simulink model "KE_time"  (Simulink 7.9)
settings: Solver=ode14x  StartTime=0.0  StopTime=6.6  FixedStep=Tsamp  RelTol=Tsamp
values from neighbouring files (symbols this model uses):
  A_hat = A_maglev    [Initialise_LQG_observers_igva.m]
  B_hat = B_maglev(:,2)    [Initialise_LQG_observers_igva.m]
  C_hat_ga = C_maglev(sensors_selected,:)    [Initialise_LQG_observers_igva.m]
  C_hat_gv = C_maglev(sensors_selected,:)    [Initialise_LQG_observers_igva.m]
  C_hat_gva = C_maglev(sensors_selected,:)    [Initialise_LQG_observers_igva.m]
  C_hat_ig = C_maglev(sensors_selected,:)    [Initialise_LQG_observers_igva.m]
  C_hat_iga = C_maglev(sensors_selected,:)    [Initialise_LQG_observers_igva.m]
  C_hat_igv = C_maglev(sensors_selected,:)    [Initialise_LQG_observers_igva.m]
  C_hat_igva = C_maglev(sensors_selected,:)    [Initialise_LQG_observers_igva.m]
  D_hat_ga = D_maglev(sensors_selected,1)    [Initialise_LQG_observers_igva.m]
  D_hat_gv = D_maglev(sensors_selected,1)    [Initialise_LQG_observers_igva.m]
  D_hat_gva = D_maglev(sensors_selected,1)    [Initialise_LQG_observers_igva.m]
  D_hat_ig = D_maglev(sensors_selected,1)    [Initialise_LQG_observers_igva.m]
  D_hat_iga = D_maglev(sensors_selected,1)    [Initialise_LQG_observers_igva.m]
  D_hat_igv = D_maglev(sensors_selected,1)    [Initialise_LQG_observers_igva.m]
  D_hat_igva = D_maglev(sensors_selected,1)    [Initialise_LQG_observers_igva.m]
  sensor_matrix_ga = sensor_matrix_full(sensors_selected,:)    [Initialise_LQG_observers_igva.m]    (also in LSDP_controllers_nntraining_data_igva.m = sensors(sensor_sele,:); initialize_LSDP_controllers_igva.m = sensors(sensor_sele,:))
  sensor_matrix_gv = sensor_matrix_full(sensors_selected,:)    [Initialise_LQG_observers_igva.m]    (also in LSDP_controllers_nntraining_data_igva.m = sensors(sensor_sele,:); initialize_LSDP_controllers_igva.m = sensors(sensor_sele,:))
  sensor_matrix_gva = sensor_matrix_full(sensors_selected,:)    [Initialise_LQG_observers_igva.m]    (also in LSDP_controllers_nntraining_data_igva.m = sensors(sensor_sele,:); initialize_LSDP_controllers_igva.m = sensors(sensor_sele,:))
  sensor_matrix_ig = sensor_matrix_full(sensors_selected,:)    [Initialise_LQG_observers_igva.m]    (also in LSDP_controllers_nntraining_data_igva.m = sensors(sensor_sele,:); initialize_LSDP_controllers_igva.m = sensors(sensor_sele,:))
  sensor_matrix_iga = sensor_matrix_full(sensors_selected,:)    [Initialise_LQG_observers_igva.m]    (also in initialize_LSDP_controllers_igva.m = sensors(sensor_sele,:))
  sensor_matrix_igv = sensor_matrix_full(sensors_selected,:)    [Initialise_LQG_observers_igva.m]    (also in LSDP_controllers_nntraining_data_igva.m = sensors(sensor_sele,:); initialize_LSDP_controllers_igva.m = sensors(sensor_sele,:))
  sensor_matrix_igva = sensors(sensor_sele,:)    [LSDP_controllers_nntraining_data_igva.m]    (also in initialize_LSDP_controllers_igva.m)
undefined symbols (not defined in the file or in its folder): Kf_lqg_ga, Kf_lqg_gv, Kf_lqg_gva, Kf_lqg_ig, Kf_lqg_iga, Kf_lqg_igv, Kf_lqg_igva
settings Model: Creator=kostas  LastModifiedBy=kostas

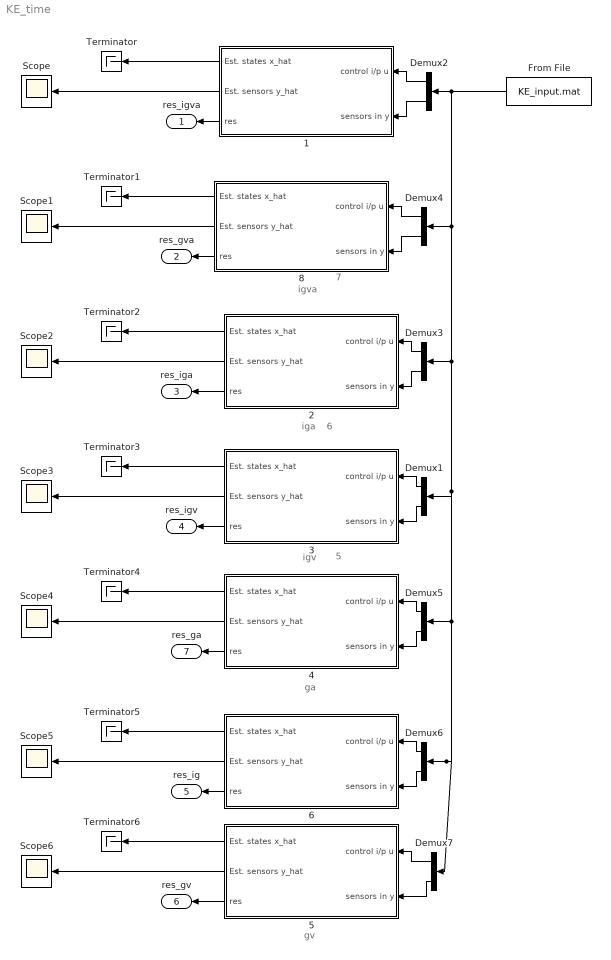
== system KE_time ==
  note: igva
  note: iga
  note: igv
  note: ga
  note: gv
  note: 7
  note: 6
  note: 5
  " 1" : Subsystem
      mask Display: fprintf('\n\n Kalman Bucy Filter \n\n (Continuous Time)\n\n')
  " 2" : Subsystem
      mask Display: fprintf('\n\n Kalman Bucy Filter \n\n (Continuous Time)\n\n')
  " 3" : Subsystem
      mask Display: fprintf('\n\n Kalman Bucy Filter \n\n (Continuous Time)\n\n')
  " 4" : Subsystem
      mask Display: fprintf('\n\n Kalman Bucy Filter \n\n (Continuous Time)\n\n')
  " 5" : Subsystem
      mask Display: fprintf('\n\n Kalman Bucy Filter \n\n (Continuous Time)\n\n')
  " 6" : Subsystem
      mask Display: fprintf('\n\n Kalman Bucy Filter \n\n (Continuous Time)\n\n')
  " 8" : Subsystem
      mask Display: fprintf('\n\n Kalman Bucy Filter \n\n (Continuous Time)\n\n')
  Demux{1..7} (7 alike) : Demux  Outputs=2
  From File : FromFile  FileName=KE_input.mat  SampleTime=0
  Scope{,1..6} (7 alike) : Scope
      Scope2 settings: SaveName=ScopeData2
      Scope3 settings: SaveName=ScopeData3
      Scope4 settings: SaveName=ScopeData4
      Scope5 settings: SaveName=ScopeData5
      Scope6 settings: SaveName=ScopeData6
  Terminator{,1..6} (7 alike) : Terminator
  res_igva : Outport
  res_gva : Outport  Port=2
  res_iga : Outport  Port=3
  res_igv : Outport  Port=4
  res_ig : Outport  Port=5
  res_gv : Outport  Port=6
  res_ga : Outport  Port=7
  wires:
  Demux2/1 -> " 1"/1(control i/p u)
  Demux2/2 -> " 1"/2(" sensors in y")
  Demux3/1 -> " 2"/1(control i/p u)
  Demux3/2 -> " 2"/2(" sensors in y")
  Demux1/1 -> " 3"/1(control i/p u)
  Demux1/2 -> " 3"/2(" sensors in y")
  Demux5/1 -> " 4"/1(control i/p u)
  Demux5/2 -> " 4"/2(" sensors in y")
  Demux6/1 -> " 6"/1(control i/p u)
  Demux6/2 -> " 6"/2(" sensors in y")
  Demux7/1 -> " 5"/1(control i/p u)
  Demux7/2 -> " 5"/2(" sensors in y")
  " 1"/3(res) -> res_igva/1
  " 2"/3(res) -> res_iga/1
  " 3"/3(res) -> res_igv/1
  " 4"/3(res) -> res_ga/1
  " 6"/3(res) -> res_ig/1
  " 5"/3(res) -> res_gv/1
  Demux4/1 -> " 8"/1(control i/p u)
  Demux4/2 -> " 8"/2(" sensors in y")
  " 8"/3(res) -> res_gva/1
  From File/1 -> Demux2/1, Demux4/1, Demux3/1, Demux5/1, Demux6/1, Demux7/1, Demux1/1
  " 1"/2(Est. sensors y_hat) -> Scope/1
  " 8"/2(Est. sensors y_hat) -> Scope1/1
  " 2"/2(Est. sensors y_hat) -> Scope2/1
  " 3"/2(Est. sensors y_hat) -> Scope3/1
  " 4"/2(Est. sensors y_hat) -> Scope4/1
  " 6"/2(Est. sensors y_hat) -> Scope5/1
  " 5"/2(Est. sensors y_hat) -> Scope6/1
  " 1"/1(Est. states x_hat) -> Terminator/1
  " 8"/1(Est. states x_hat) -> Terminator1/1
  " 2"/1(Est. states x_hat) -> Terminator2/1
  " 3"/1(Est. states x_hat) -> Terminator3/1
  " 4"/1(Est. states x_hat) -> Terminator4/1
  " 6"/1(Est. states x_hat) -> Terminator5/1
  " 5"/1(Est. states x_hat) -> Terminator6/1

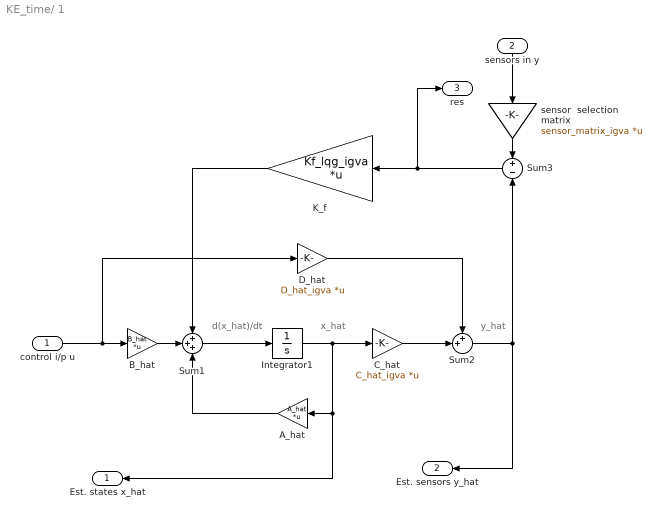
== system KE_time/ 1 ==
  note: d(x_hat)/dt
  note: x_hat
  note: y_hat
  control i/p u : Inport
  " sensors in y" : Inport  Port=2
  "A_hat " : Gain  Gain=A_hat  Multiplication=Matrix(K*u)  SaturateOnIntegerOverflow=on  OutDataTypeStr=Inherit: Same as input  ParamDataTypeStr=Inherit: Same as input
  B_hat : Gain  Gain=B_hat  Multiplication=Matrix(K*u)  SaturateOnIntegerOverflow=on  OutDataTypeStr=Inherit: Same as input  ParamDataTypeStr=Inherit: Same as input
  C_hat : Gain  Gain=C_hat_igva  Multiplication=Matrix(K*u)  SaturateOnIntegerOverflow=on  OutDataTypeStr=Inherit: Same as input  ParamDataTypeStr=Inherit: Same as input
  D_hat : Gain  Gain=D_hat_igva  Multiplication=Matrix(K*u)  SaturateOnIntegerOverflow=on  OutDataTypeStr=Inherit: Same as input  ParamDataTypeStr=Inherit: Same as input
  Integrator1 : Integrator
  K_f : Gain  Gain=Kf_lqg_igva  Multiplication=Matrix(K*u)  SaturateOnIntegerOverflow=on  OutDataTypeStr=Inherit: Same as input  ParamDataTypeStr=Inherit: Same as input
  Sum1 : Sum  Inputs=+++  SaturateOnIntegerOverflow=on  InputSameDT=on  OutDataTypeStr=Inherit: Same as first input
  Sum2 : Sum  Inputs=++|  SaturateOnIntegerOverflow=on  InputSameDT=on  OutDataTypeStr=Inherit: Same as first input
  Sum3 : Sum  Inputs=+|-  SaturateOnIntegerOverflow=on  InputSameDT=on  OutDataTypeStr=Inherit: Same as first input
  sensor  selection  matrix : Gain  Gain=sensor_matrix_igva  Multiplication=Matrix(K*u) (u vector)
  Est. states x_hat : Outport  OutputWhenDisabled=reset  InitialOutput=[0 0 0]
  Est. sensors y_hat : Outport  Port=2
  res : Outport  Port=3
  wires:
  Sum2/1 -> Est. sensors y_hat/1, Sum3/2
  D_hat/1 -> Sum2/1
  C_hat/1 -> Sum2/2
  control i/p u/1 -> D_hat/1, B_hat/1
  " sensors in y"/1 -> sensor  selection  matrix/1
  Sum3/1 -> K_f/1, res/1
  K_f/1 -> Sum1/1
  Integrator1/1 -> Est. states x_hat/1, "A_hat "/1, C_hat/1
  Sum1/1 -> Integrator1/1
  "A_hat "/1 -> Sum1/3
  B_hat/1 -> Sum1/2
  sensor  selection  matrix/1 -> Sum3/1

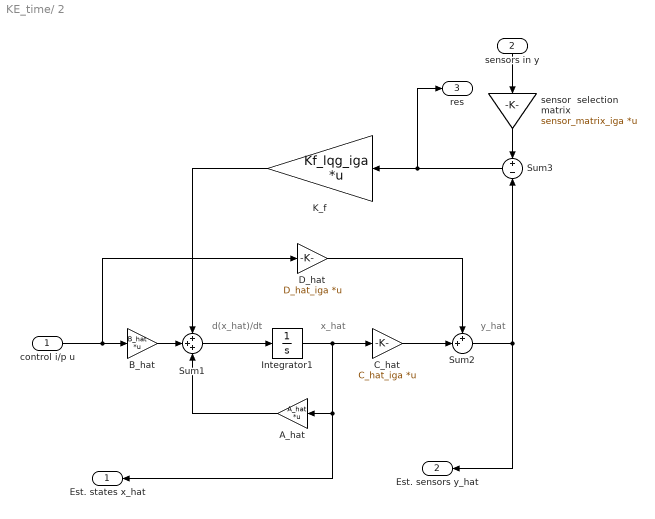
== system KE_time/ 2 ==
  note: y_hat
  note: x_hat
  note: d(x_hat)/dt
  control i/p u : Inport
  " sensors in y" : Inport  Port=2
  "A_hat " : Gain  Gain=A_hat  Multiplication=Matrix(K*u)  SaturateOnIntegerOverflow=on  OutDataTypeStr=Inherit: Same as input  ParamDataTypeStr=Inherit: Same as input
  B_hat : Gain  Gain=B_hat  Multiplication=Matrix(K*u)  SaturateOnIntegerOverflow=on  OutDataTypeStr=Inherit: Same as input  ParamDataTypeStr=Inherit: Same as input
  C_hat : Gain  Gain=C_hat_iga  Multiplication=Matrix(K*u)  SaturateOnIntegerOverflow=on  OutDataTypeStr=Inherit: Same as input  ParamDataTypeStr=Inherit: Same as input
  D_hat : Gain  Gain=D_hat_iga  Multiplication=Matrix(K*u)  SaturateOnIntegerOverflow=on  OutDataTypeStr=Inherit: Same as input  ParamDataTypeStr=Inherit: Same as input
  Integrator1 : Integrator
  K_f : Gain  Gain=Kf_lqg_iga  Multiplication=Matrix(K*u)  SaturateOnIntegerOverflow=on  OutDataTypeStr=Inherit: Same as input  ParamDataTypeStr=Inherit: Same as input
  Sum1 : Sum  Inputs=+++  SaturateOnIntegerOverflow=on  InputSameDT=on  OutDataTypeStr=Inherit: Same as first input
  Sum2 : Sum  Inputs=++|  SaturateOnIntegerOverflow=on  InputSameDT=on  OutDataTypeStr=Inherit: Same as first input
  Sum3 : Sum  Inputs=+|-  SaturateOnIntegerOverflow=on  InputSameDT=on  OutDataTypeStr=Inherit: Same as first input
  sensor  selection  matrix : Gain  Gain=sensor_matrix_iga  Multiplication=Matrix(K*u) (u vector)
  Est. states x_hat : Outport  OutputWhenDisabled=reset  InitialOutput=[0 0 0]
  Est. sensors y_hat : Outport  Port=2
  res : Outport  Port=3
  wires:
  sensor  selection  matrix/1 -> Sum3/1
  B_hat/1 -> Sum1/2
  "A_hat "/1 -> Sum1/3
  Sum1/1 -> Integrator1/1
  Integrator1/1 -> C_hat/1, "A_hat "/1, Est. states x_hat/1
  K_f/1 -> Sum1/1
  Sum3/1 -> K_f/1, res/1
  " sensors in y"/1 -> sensor  selection  matrix/1
  control i/p u/1 -> B_hat/1, D_hat/1
  C_hat/1 -> Sum2/2
  D_hat/1 -> Sum2/1
  Sum2/1 -> Sum3/2, Est. sensors y_hat/1

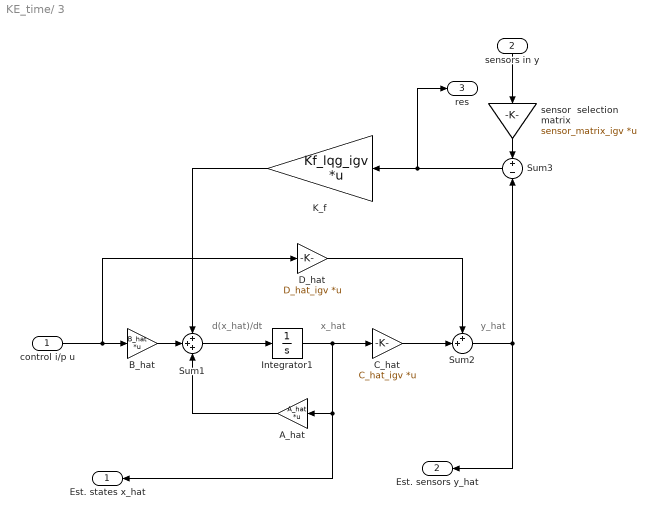
== system KE_time/ 3 ==
  note: d(x_hat)/dt
  note: x_hat
  note: y_hat
  control i/p u : Inport
  " sensors in y" : Inport  Port=2
  "A_hat " : Gain  Gain=A_hat  Multiplication=Matrix(K*u)  SaturateOnIntegerOverflow=on  OutDataTypeStr=Inherit: Same as input  ParamDataTypeStr=Inherit: Same as input
  B_hat : Gain  Gain=B_hat  Multiplication=Matrix(K*u)  SaturateOnIntegerOverflow=on  OutDataTypeStr=Inherit: Same as input  ParamDataTypeStr=Inherit: Same as input
  C_hat : Gain  Gain=C_hat_igv  Multiplication=Matrix(K*u)  SaturateOnIntegerOverflow=on  OutDataTypeStr=Inherit: Same as input  ParamDataTypeStr=Inherit: Same as input
  D_hat : Gain  Gain=D_hat_igv  Multiplication=Matrix(K*u)  SaturateOnIntegerOverflow=on  OutDataTypeStr=Inherit: Same as input  ParamDataTypeStr=Inherit: Same as input
  Integrator1 : Integrator
  K_f : Gain  Gain=Kf_lqg_igv  Multiplication=Matrix(K*u)  SaturateOnIntegerOverflow=on  OutDataTypeStr=Inherit: Same as input  ParamDataTypeStr=Inherit: Same as input
  Sum1 : Sum  Inputs=+++  SaturateOnIntegerOverflow=on  InputSameDT=on  OutDataTypeStr=Inherit: Same as first input
  Sum2 : Sum  Inputs=++|  SaturateOnIntegerOverflow=on  InputSameDT=on  OutDataTypeStr=Inherit: Same as first input
  Sum3 : Sum  Inputs=+|-  SaturateOnIntegerOverflow=on  InputSameDT=on  OutDataTypeStr=Inherit: Same as first input
  sensor  selection  matrix : Gain  Gain=sensor_matrix_igv  Multiplication=Matrix(K*u) (u vector)
  Est. states x_hat : Outport  OutputWhenDisabled=reset  InitialOutput=[0 0 0]
  Est. sensors y_hat : Outport  Port=2
  res : Outport  Port=3
  wires:
  Sum2/1 -> Est. sensors y_hat/1, Sum3/2
  D_hat/1 -> Sum2/1
  C_hat/1 -> Sum2/2
  control i/p u/1 -> D_hat/1, B_hat/1
  " sensors in y"/1 -> sensor  selection  matrix/1
  Sum3/1 -> res/1, K_f/1
  K_f/1 -> Sum1/1
  Integrator1/1 -> Est. states x_hat/1, "A_hat "/1, C_hat/1
  Sum1/1 -> Integrator1/1
  "A_hat "/1 -> Sum1/3
  B_hat/1 -> Sum1/2
  sensor  selection  matrix/1 -> Sum3/1

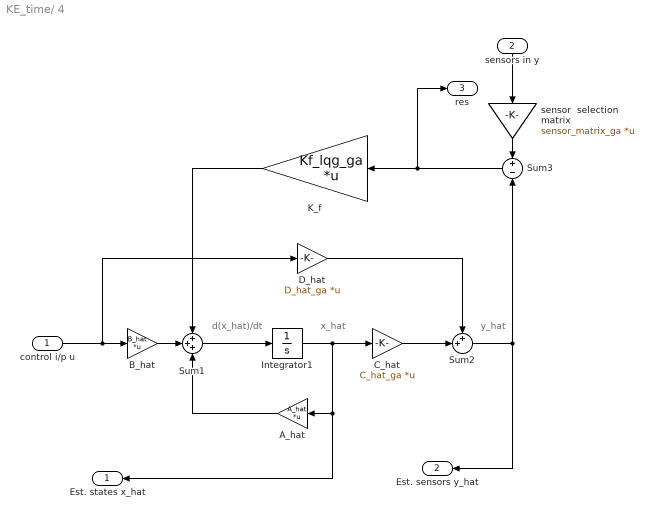
== system KE_time/ 4 ==
  note: y_hat
  note: x_hat
  note: d(x_hat)/dt
  control i/p u : Inport
  " sensors in y" : Inport  Port=2
  "A_hat " : Gain  Gain=A_hat  Multiplication=Matrix(K*u)  SaturateOnIntegerOverflow=on  OutDataTypeStr=Inherit: Same as input  ParamDataTypeStr=Inherit: Same as input
  B_hat : Gain  Gain=B_hat  Multiplication=Matrix(K*u)  SaturateOnIntegerOverflow=on  OutDataTypeStr=Inherit: Same as input  ParamDataTypeStr=Inherit: Same as input
  C_hat : Gain  Gain=C_hat_ga  Multiplication=Matrix(K*u)  SaturateOnIntegerOverflow=on  OutDataTypeStr=Inherit: Same as input  ParamDataTypeStr=Inherit: Same as input
  D_hat : Gain  Gain=D_hat_ga  Multiplication=Matrix(K*u)  SaturateOnIntegerOverflow=on  OutDataTypeStr=Inherit: Same as input  ParamDataTypeStr=Inherit: Same as input
  Integrator1 : Integrator
  K_f : Gain  Gain=Kf_lqg_ga  Multiplication=Matrix(K*u)  SaturateOnIntegerOverflow=on  OutDataTypeStr=Inherit: Same as input  ParamDataTypeStr=Inherit: Same as input
  Sum1 : Sum  Inputs=+++  SaturateOnIntegerOverflow=on  InputSameDT=on  OutDataTypeStr=Inherit: Same as first input
  Sum2 : Sum  Inputs=++|  SaturateOnIntegerOverflow=on  InputSameDT=on  OutDataTypeStr=Inherit: Same as first input
  Sum3 : Sum  Inputs=+|-  SaturateOnIntegerOverflow=on  InputSameDT=on  OutDataTypeStr=Inherit: Same as first input
  sensor  selection  matrix : Gain  Gain=sensor_matrix_ga  Multiplication=Matrix(K*u) (u vector)
  Est. states x_hat : Outport  OutputWhenDisabled=reset  InitialOutput=[0 0 0]
  Est. sensors y_hat : Outport  Port=2
  res : Outport  Port=3
  wires:
  sensor  selection  matrix/1 -> Sum3/1
  B_hat/1 -> Sum1/2
  "A_hat "/1 -> Sum1/3
  Sum1/1 -> Integrator1/1
  Integrator1/1 -> C_hat/1, "A_hat "/1, Est. states x_hat/1
  K_f/1 -> Sum1/1
  Sum3/1 -> K_f/1, res/1
  " sensors in y"/1 -> sensor  selection  matrix/1
  control i/p u/1 -> B_hat/1, D_hat/1
  C_hat/1 -> Sum2/2
  D_hat/1 -> Sum2/1
  Sum2/1 -> Sum3/2, Est. sensors y_hat/1

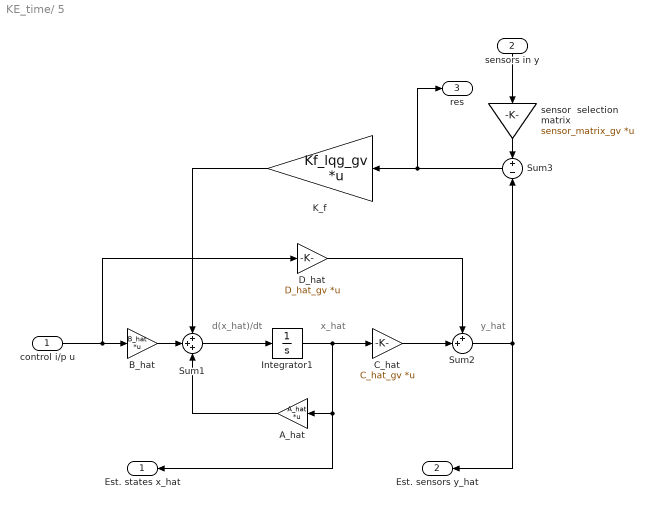
== system KE_time/ 5 ==
  note: d(x_hat)/dt
  note: x_hat
  note: y_hat
  control i/p u : Inport
  " sensors in y" : Inport  Port=2
  "A_hat " : Gain  Gain=A_hat  Multiplication=Matrix(K*u)  SaturateOnIntegerOverflow=on  OutDataTypeStr=Inherit: Same as input  ParamDataTypeStr=Inherit: Same as input
  B_hat : Gain  Gain=B_hat  Multiplication=Matrix(K*u)  SaturateOnIntegerOverflow=on  OutDataTypeStr=Inherit: Same as input  ParamDataTypeStr=Inherit: Same as input
  C_hat : Gain  Gain=C_hat_gv  Multiplication=Matrix(K*u)  SaturateOnIntegerOverflow=on  OutDataTypeStr=Inherit: Same as input  ParamDataTypeStr=Inherit: Same as input
  D_hat : Gain  Gain=D_hat_gv  Multiplication=Matrix(K*u)  SaturateOnIntegerOverflow=on  OutDataTypeStr=Inherit: Same as input  ParamDataTypeStr=Inherit: Same as input
  Integrator1 : Integrator
  K_f : Gain  Gain=Kf_lqg_gv  Multiplication=Matrix(K*u)  SaturateOnIntegerOverflow=on  OutDataTypeStr=Inherit: Same as input  ParamDataTypeStr=Inherit: Same as input
  Sum1 : Sum  Inputs=+++  SaturateOnIntegerOverflow=on  InputSameDT=on  OutDataTypeStr=Inherit: Same as first input
  Sum2 : Sum  Inputs=++|  SaturateOnIntegerOverflow=on  InputSameDT=on  OutDataTypeStr=Inherit: Same as first input
  Sum3 : Sum  Inputs=+|-  SaturateOnIntegerOverflow=on  InputSameDT=on  OutDataTypeStr=Inherit: Same as first input
  sensor  selection  matrix : Gain  Gain=sensor_matrix_gv  Multiplication=Matrix(K*u) (u vector)
  Est. states x_hat : Outport  OutputWhenDisabled=reset  InitialOutput=[0 0 0]
  Est. sensors y_hat : Outport  Port=2
  res : Outport  Port=3
  wires:
  Sum2/1 -> Est. sensors y_hat/1, Sum3/2
  D_hat/1 -> Sum2/1
  C_hat/1 -> Sum2/2
  control i/p u/1 -> D_hat/1, B_hat/1
  " sensors in y"/1 -> sensor  selection  matrix/1
  Sum3/1 -> res/1, K_f/1
  K_f/1 -> Sum1/1
  Integrator1/1 -> Est. states x_hat/1, "A_hat "/1, C_hat/1
  Sum1/1 -> Integrator1/1
  "A_hat "/1 -> Sum1/3
  B_hat/1 -> Sum1/2
  sensor  selection  matrix/1 -> Sum3/1

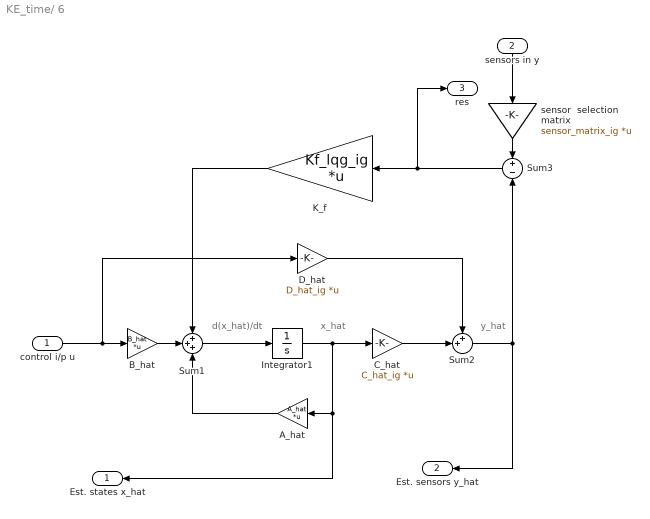
== system KE_time/ 6 ==
  note: y_hat
  note: x_hat
  note: d(x_hat)/dt
  control i/p u : Inport
  " sensors in y" : Inport  Port=2
  "A_hat " : Gain  Gain=A_hat  Multiplication=Matrix(K*u)  SaturateOnIntegerOverflow=on  OutDataTypeStr=Inherit: Same as input  ParamDataTypeStr=Inherit: Same as input
  B_hat : Gain  Gain=B_hat  Multiplication=Matrix(K*u)  SaturateOnIntegerOverflow=on  OutDataTypeStr=Inherit: Same as input  ParamDataTypeStr=Inherit: Same as input
  C_hat : Gain  Gain=C_hat_ig  Multiplication=Matrix(K*u)  SaturateOnIntegerOverflow=on  OutDataTypeStr=Inherit: Same as input  ParamDataTypeStr=Inherit: Same as input
  D_hat : Gain  Gain=D_hat_ig  Multiplication=Matrix(K*u)  SaturateOnIntegerOverflow=on  OutDataTypeStr=Inherit: Same as input  ParamDataTypeStr=Inherit: Same as input
  Integrator1 : Integrator
  K_f : Gain  Gain=Kf_lqg_ig  Multiplication=Matrix(K*u)  SaturateOnIntegerOverflow=on  OutDataTypeStr=Inherit: Same as input  ParamDataTypeStr=Inherit: Same as input
  Sum1 : Sum  Inputs=+++  SaturateOnIntegerOverflow=on  InputSameDT=on  OutDataTypeStr=Inherit: Same as first input
  Sum2 : Sum  Inputs=++|  SaturateOnIntegerOverflow=on  InputSameDT=on  OutDataTypeStr=Inherit: Same as first input
  Sum3 : Sum  Inputs=+|-  SaturateOnIntegerOverflow=on  InputSameDT=on  OutDataTypeStr=Inherit: Same as first input
  sensor  selection  matrix : Gain  Gain=sensor_matrix_ig  Multiplication=Matrix(K*u) (u vector)
  Est. states x_hat : Outport  OutputWhenDisabled=reset  InitialOutput=[0 0 0]
  Est. sensors y_hat : Outport  Port=2
  res : Outport  Port=3
  wires:
  sensor  selection  matrix/1 -> Sum3/1
  B_hat/1 -> Sum1/2
  "A_hat "/1 -> Sum1/3
  Sum1/1 -> Integrator1/1
  Integrator1/1 -> C_hat/1, "A_hat "/1, Est. states x_hat/1
  K_f/1 -> Sum1/1
  Sum3/1 -> K_f/1, res/1
  " sensors in y"/1 -> sensor  selection  matrix/1
  control i/p u/1 -> B_hat/1, D_hat/1
  C_hat/1 -> Sum2/2
  D_hat/1 -> Sum2/1
  Sum2/1 -> Sum3/2, Est. sensors y_hat/1

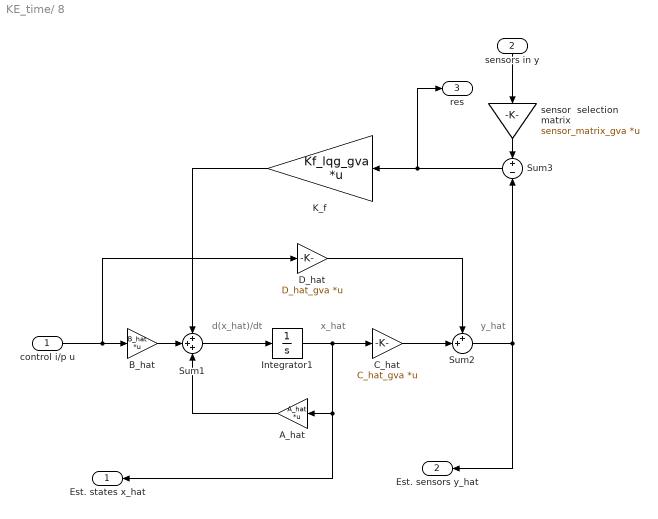
== system KE_time/ 8 ==
  note: y_hat
  note: x_hat
  note: d(x_hat)/dt
  control i/p u : Inport
  " sensors in y" : Inport  Port=2
  "A_hat " : Gain  Gain=A_hat  Multiplication=Matrix(K*u)  SaturateOnIntegerOverflow=on  OutDataTypeStr=Inherit: Same as input  ParamDataTypeStr=Inherit: Same as input
  B_hat : Gain  Gain=B_hat  Multiplication=Matrix(K*u)  SaturateOnIntegerOverflow=on  OutDataTypeStr=Inherit: Same as input  ParamDataTypeStr=Inherit: Same as input
  C_hat : Gain  Gain=C_hat_gva  Multiplication=Matrix(K*u)  SaturateOnIntegerOverflow=on  OutDataTypeStr=Inherit: Same as input  ParamDataTypeStr=Inherit: Same as input
  D_hat : Gain  Gain=D_hat_gva  Multiplication=Matrix(K*u)  SaturateOnIntegerOverflow=on  OutDataTypeStr=Inherit: Same as input  ParamDataTypeStr=Inherit: Same as input
  Integrator1 : Integrator
  K_f : Gain  Gain=Kf_lqg_gva  Multiplication=Matrix(K*u)  SaturateOnIntegerOverflow=on  OutDataTypeStr=Inherit: Same as input  ParamDataTypeStr=Inherit: Same as input
  Sum1 : Sum  Inputs=+++  SaturateOnIntegerOverflow=on  InputSameDT=on  OutDataTypeStr=Inherit: Same as first input
  Sum2 : Sum  Inputs=++|  SaturateOnIntegerOverflow=on  InputSameDT=on  OutDataTypeStr=Inherit: Same as first input
  Sum3 : Sum  Inputs=+|-  SaturateOnIntegerOverflow=on  InputSameDT=on  OutDataTypeStr=Inherit: Same as first input
  sensor  selection  matrix : Gain  Gain=sensor_matrix_gva  Multiplication=Matrix(K*u) (u vector)
  Est. states x_hat : Outport  OutputWhenDisabled=reset  InitialOutput=[0 0 0]
  Est. sensors y_hat : Outport  Port=2
  res : Outport  Port=3
  wires:
  sensor  selection  matrix/1 -> Sum3/1
  B_hat/1 -> Sum1/2
  "A_hat "/1 -> Sum1/3
  Sum1/1 -> Integrator1/1
  Integrator1/1 -> C_hat/1, "A_hat "/1, Est. states x_hat/1
  K_f/1 -> Sum1/1
  Sum3/1 -> res/1, K_f/1
  " sensors in y"/1 -> sensor  selection  matrix/1
  control i/p u/1 -> B_hat/1, D_hat/1
  C_hat/1 -> Sum2/2
  D_hat/1 -> Sum2/1
  Sum2/1 -> Sum3/2, Est. sensors y_hat/1
